simulink model "non_linear_tank_system_control101"  (R2023b)
settings: Solver=ode45  StartTime=0.0  StopTime=endtime  RelTol=1e-3  EnableMultiTasking=on
undefined symbols (not defined in the file): Ai, Aie, blockagetime, C, Cl, Ctemp, hss, hsse, qchangetime, qss, qsse, qstep
settings Model: Creator=stelios  LastModifiedBy=Anthony Rossiter
settings DataIOCC: LimitDataPoints=on  SaveFormat=Array  SignalLoggingSaveFormat=ModelDataLogs  ReturnWorkspaceOutputs=off
settings OptimizationCC: BooleanDataType=off
settings DebuggingCC: SaveWithParameterizedLinksMsg=none  UnderspecifiedInitializationDetection=Classic  MergeDetectMultiDrivingBlocksExec=none  SignalResolutionControl=TryResolveAllWithWarning  InheritedTsInSrcMsg=none  MultiTaskDSMMsg=warning  MultiTaskCondExecSysMsg=none  UnconnectedInputMsg=warning  UnconnectedOutputMsg=warning  UnconnectedLineMsg=warning
settings HardwareCC: TargetUnknown=on
settings ModelReferenceCC: EnableRefExpFcnMdlSchedulingChecks=on  PropagateSignalLabelsOutOfModel=off
settings RTWCC: DLArmComputeVersion=19.05
settings GRTTargetCC: CombineOutputUpdateFcns=off  GRTInterface=on
settings ConfigComp: CovMetricSettings=dw

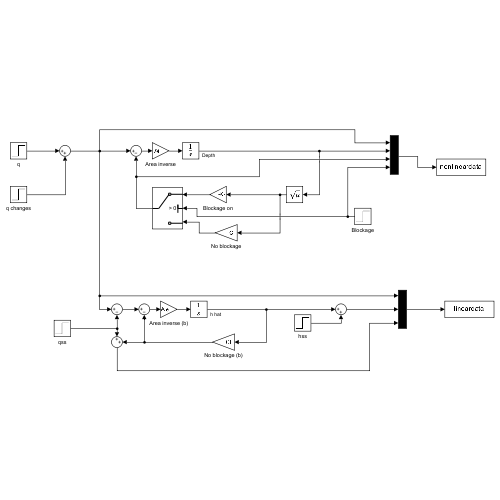
[thumbnail: Simulink's stored preview of the top-level diagram]
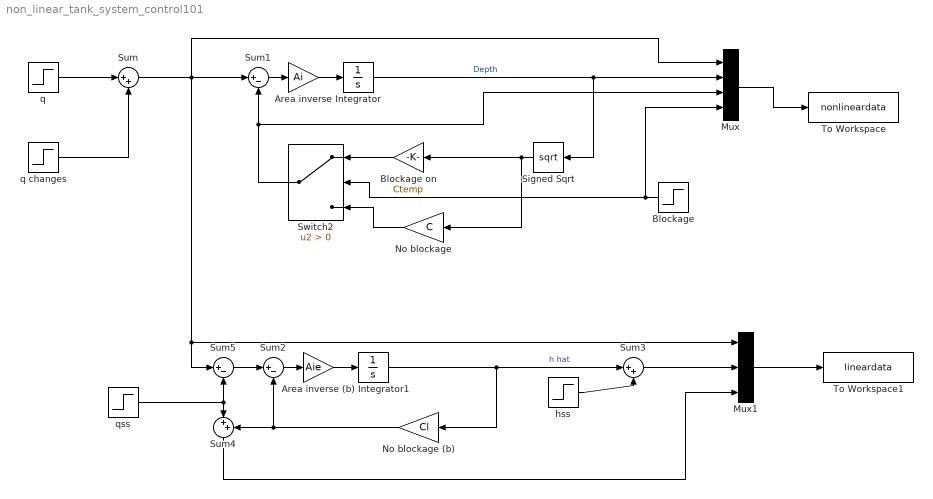
== system non_linear_tank_system_control101 ==
  Area inverse : Gain  Gain=Ai  SaturateOnIntegerOverflow=on
  Area inverse (b) : Gain  Gain=Aie  SaturateOnIntegerOverflow=on
  Blockage : Step  Time=blockagetime
  Blockage on : Gain  Gain=Ctemp  SaturateOnIntegerOverflow=on
  Integrator : Integrator  InitialCondition=hss
  Integrator1 : Integrator
  Mux : Mux
  Mux1 : Mux  Inputs=3
  No blockage : Gain  Gain=C  SaturateOnIntegerOverflow=on
  No blockage (b) : Gain  Gain=Cl  SaturateOnIntegerOverflow=on
  Signed Sqrt : Sqrt
  Sum : Sum  Inputs=|++
  Sum1 : Sum  Inputs=|+-  SaturateOnIntegerOverflow=on
  Sum2 : Sum  Inputs=|+-  SaturateOnIntegerOverflow=on
  Sum3 : Sum  Inputs=|++
  Sum4 : Sum  Inputs=|++
  Sum5 : Sum  Inputs=|+-
  Switch2 : Switch  Criteria=u2 > Threshold  SaturateOnIntegerOverflow=off  InputSameDT=off
  To Workspace : ToWorkspace  VariableName=nonlineardata  SaveFormat=Structure With Time  SampleTime=-1
  To Workspace1 : ToWorkspace  VariableName=lineardata  SaveFormat=Structure With Time  SampleTime=-1
  hss : Step  Time=0.2  After=hsse
  q : Step  Time=0  After=qss
  q changes : Step  Time=qchangetime  After=qstep
  qss : Step  Time=0.2  After=qsse
  wires:
  Mux/1 -> To Workspace/1
  Signed Sqrt/1 -> No blockage/1, Blockage on/1
  Integrator/1 -> Signed Sqrt/1, Mux/2  "Depth"
  Sum1/1 -> Area inverse/1
  Blockage on/1 -> Switch2/1
  No blockage/1 -> Switch2/3
  Blockage/1 -> Mux/4, Switch2/2
  Switch2/1 -> Mux/3, Sum1/2
  Area inverse/1 -> Integrator/1
  Sum2/1 -> Area inverse (b)/1
  Mux1/1 -> To Workspace1/1
  Area inverse (b)/1 -> Integrator1/1
  Integrator1/1 -> No blockage (b)/1, Sum3/1  "h hat"
  Sum5/1 -> Sum2/1
  qss/1 -> Sum4/1, Sum5/2
  Sum3/1 -> Mux1/2
  hss/1 -> Sum3/2
  No blockage (b)/1 -> Sum4/2, Sum2/2
  Sum/1 -> Mux1/1, Sum5/1, Mux/1, Sum1/1
  q/1 -> Sum/1
  q changes/1 -> Sum/2
  Sum4/1 -> Mux1/3
